simulink library "steadyLevelFlightController_cl"  (R2020a)
settings: Solver=VariableStepAuto  StartTime=0.0  StopTime=10.0  RelTol=1e-3
undefined symbols (not defined in the file or in its folder): env, FLIGHTCONTROLLER, fltCtrl, initializeBussesFromBlock, vhcl
libraries: filteredPIDController_ul x4, ctrlAllocMatrix_cl x1, eulAng2RotMat_ul x1, alphaBeta_ul x1, gnd2TanRotation_ul x1
settings Model: Creator=jldanie5  LastModifiedBy=John Jr
settings DataIOCC: ReturnWorkspaceOutputs=off
settings DebuggingCC: ArithmeticOperatorsInVariantConditions=warning
settings SFSimCC: CustomCodeUndefinedFunction=UseInterfaceOnly

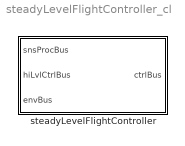
== system steadyLevelFlightController_cl ==
  steadyLevelFlightController : Subsystem  LoadFcn=initializeBussesFromBlock(gcb)  InitFcn=initializeBussesFromBlock(gcb)  StartFcn=initializeBussesFromBlock(gcb)  VariantControl=strcmpi(FLIGHTCONTROLLER,'steadyLevelFlightController')  mask{initPosForInitSStar=vhcl.initPosVecGnd.Value, fluidDensity=env.water.density.Value, pathCtrl=fltCtrl, aeroStruct=vhcl.struct('OCT.aeroSurf')}
      mask prompts: initPosForInitSStar "Initial Position"; fluidDensity "Fluid Density"; pathCtrl "Controller"; aeroStruct "Aerodynamic Structure"
      settings: MinAlgLoopOccurrences=on
      mask DialogControl Container3 Prompt: courseFollow Params
      mask DialogControl Container4 Prompt: setpointToOutput Params

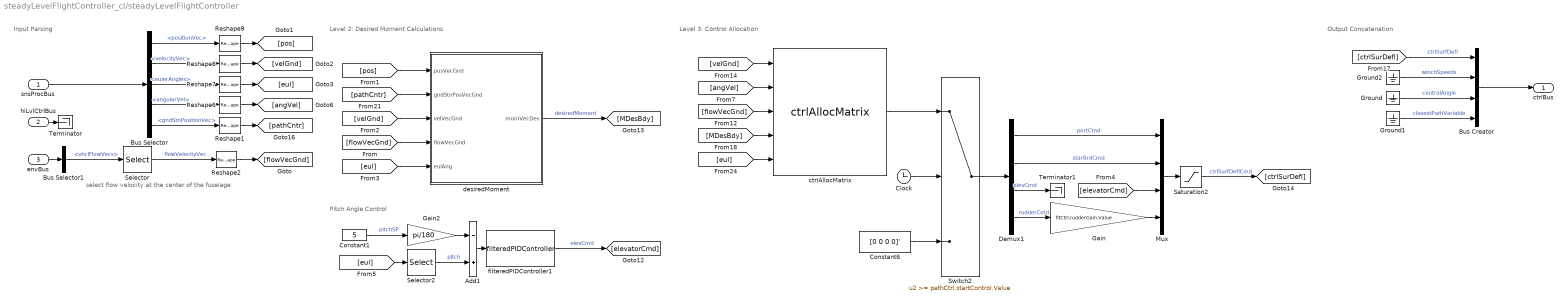
== system steadyLevelFlightController_cl/steadyLevelFlightController ==
  note: select flow velocity at the center of the fuselage
  note: Level 3: Control Allocation
  note: Output Concatenation
  note: Level 2: Desired Moment Calculations
  note: Input Parsing
  note: Pitch Angle Control
  snsProcBus : Inport  OutDataTypeStr=Bus: sensorsProcessingBus
  hiLvlCtrlBus : Inport  Port=2  OutDataTypeStr=Bus: hiLvlCtrlBus
  envBus : Inport  Port=3  OutDataTypeStr=Bus: envBus
  Add1 : Sum  Inputs=-+
  Bus Creator : BusCreator  Inputs=4  OutDataTypeStr=Bus: fltCtrlBus
      settings: InheritFromInputs=off
  Bus Selector : BusSelector  OutputSignals=positionVec,velocityVec,eulerAngles,angularVel,gndStnPositionVec
  Bus Selector1 : BusSelector  OutputSignals=vhclFlowVecs
  Clock : Clock
  Constant1 : Constant  Value=5
  Constant6 : Constant  Value=[0 0 0 0]'
  Demux1 : Demux
  Gain : Gain  Gain=fltCtrl.rudderGain.Value
  Gain2 : Gain  Gain=pi/180
  Ground : Ground
  Ground1 : Ground
  Ground2 : Ground
  Mux : Mux
  Reshape{1..2,6..9} (6 alike) : Reshape  OutputDimensionality=Column vector (2-D)
  Saturation2 : Saturate  UpperLimit=pathCtrl.controlSigMax.upperLimit.Value  LowerLimit=pathCtrl.controlSigMax.lowerLimit.Value
  Selector : Selector  NumberOfDimensions=2  InputPortWidth=3  IndexOptions=Select all,Index vector (dialog)  Indices=[1 3],5  OutputSizes=1,1
  Selector2 : Selector  InputPortWidth=3  IndexOptions=Index vector (dialog)  Indices=2  OutputSizes=1
  Switch2 : Switch  Threshold=pathCtrl.startControl.Value
  Terminator : Terminator
  Terminator1 : Terminator
  ctrlAllocMatrix : ctrlAllocMatrix_cl/ctrlAllocMatrix  aeroStruct=aeroStruct  fluidDensity=fluidDensity
  desiredMoment : Subsystem
  filteredPIDController1 : filteredPIDController_ul/filteredPIDController  kp=pathCtrl.pitchMoment.kp.Value  ki=pathCtrl.pitchMoment.ki.Value  kd=pathCtrl.pitchMoment.kd.Value  Value=pathCtrl.pitchMoment.tau.Value  externalReset=none
  ctrlBus : Outport  OutDataTypeStr=Bus: fltCtrlBus  VectorParamsAs1DForOutWhenUnconnected=off
  wires:
  snsProcBus/1 -> Bus Selector/1
  Bus Selector/2 -> Reshape8/1  "<velocityVec>"
  Bus Selector/1 -> Reshape9/1  "<positionVec>"
  Bus Selector/3 -> Reshape7/1  "<eulerAngles>"
  Bus Creator/1 -> ctrlBus/1
  Ground2/1 -> Bus Creator/2  "winchSpeeds"
  Ground/1 -> Bus Creator/3  "centralAngle"
  Ground1/1 -> Bus Creator/4  "closestPathVariable"
  desiredMoment/1(momVecDes) -> [MDesBdy]  "desiredMoment"
  Bus Selector/4 -> Reshape6/1  "<angularVel>"
  [angVel] -> ctrlAllocMatrix/2
  [velGnd] -> ctrlAllocMatrix/1
  [flowVecGnd] -> ctrlAllocMatrix/3
  Demux1/1 -> Mux/1  "portCmd"
  Demux1/2 -> Mux/2  "starBrdCmd"
  Clock/1 -> Switch2/2
  Switch2/1 -> Demux1/1
  Constant6/1 -> Switch2/3
  [MDesBdy] -> ctrlAllocMatrix/4
  ctrlAllocMatrix/1 -> Switch2/1
  [ctrlSurDefl] -> Bus Creator/1  "ctrlSurfDefl"
  Saturation2/1 -> [ctrlSurDefl]  "ctrlSurfDeflCmd"
  Reshape2/1 -> [flowVecGnd]
  Reshape6/1 -> [angVel]
  Reshape7/1 -> [eul]
  Reshape8/1 -> [velGnd]
  Reshape9/1 -> [pos]
  [eul] -> ctrlAllocMatrix/5
  Selector/1 -> Reshape2/1  "flowVelocityVec"
  envBus/1 -> Bus Selector1/1
  Bus Selector1/1 -> Selector/1  "<vhclFlowVecs>"
  Reshape1/1 -> [pathCntr]
  Bus Selector/5 -> Reshape1/1  "<gndStnPositionVec>"
  [pos] -> desiredMoment/1(posVecGnd)
  [pathCntr] -> desiredMoment/2(gndStnPosVecGnd)
  [velGnd] -> desiredMoment/3(velVecGnd)
  [eul] -> desiredMoment/5(eulAng)
  [flowVecGnd] -> desiredMoment/4(flowVecGnd)
  Gain/1 -> Mux/4
  Demux1/4 -> Gain/1  "rudderCmd"
  hiLvlCtrlBus/1 -> Terminator/1
  Mux/1 -> Saturation2/1
  Demux1/3 -> Terminator1/1  "elevCmd"
  Gain2/1 -> Add1/1
  [eul] -> Selector2/1
  Add1/1 -> filteredPIDController1/1
  Selector2/1 -> Add1/2  "pitch"
  Constant1/1 -> Gain2/1  "pitchSP"
  filteredPIDController1/1 -> [elevatorCmd]  "elevCmd"
  [elevatorCmd] -> Mux/3

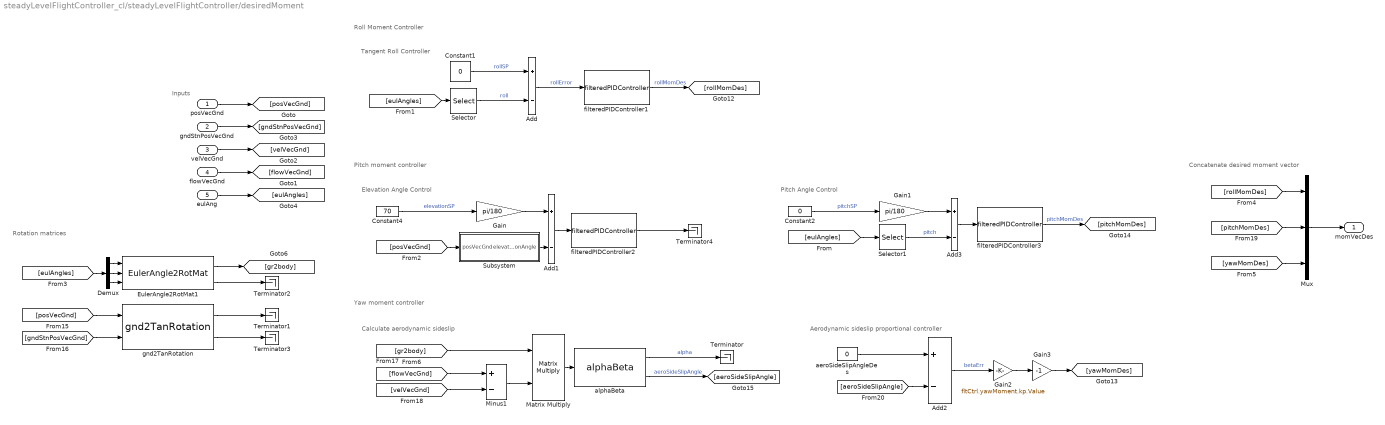
== system steadyLevelFlightController_cl/steadyLevelFlightController/desiredMoment ==
  note: Elevation Angle Control
  note: Inputs
  note: Rotation matrices
  note: Tangent Roll Controller
  note: Concatenate desired moment vector
  note: Aerodynamic sideslip proportional controller
  note: Calculate aerodynamic sideslip
  note: Yaw moment controller
  note: Pitch moment controller
  note: Roll Moment Controller
  note: Pitch Angle Control
  posVecGnd : Inport
  gndStnPosVecGnd : Inport  Port=2
  velVecGnd : Inport  Port=3
  flowVecGnd : Inport  Port=4
  eulAng : Inport  Port=5
  Add{,1..3} (4 alike) : Sum  Inputs=+-
  Constant1 : Constant  Value=0
  Constant2 : Constant  Value=0
  Constant4 : Constant  Value=70
  Demux : Demux  Outputs=3
  EulerAngle2RotMat1 : eulAng2RotMat_ul/EulerAngle2RotMat  SystemSampleTime=-1  Latency=0  AutoFrameSizeCalculation=off
  Gain : Gain  Gain=pi/180
  Gain1 : Gain  Gain=pi/180
  Gain2 : Gain  Gain=fltCtrl.yawMoment.kp.Value
  Gain3 : Gain  Gain=-1
  Matrix Multiply : Product  Multiplication=Matrix(*)
  Minus1 : Sum  Inputs=+-
  Mux : Mux  Inputs=3
  Selector : Selector  InputPortWidth=3  IndexOptions=Index vector (dialog)  Indices=1  OutputSizes=1
  Selector1 : Selector  InputPortWidth=3  IndexOptions=Index vector (dialog)  Indices=2  OutputSizes=1
  Subsystem : Subsystem
  Terminator{,1..4} (5 alike) : Terminator
  aeroSideSlipAngleDes : Constant  Value=0
  alphaBeta : alphaBeta_ul/alphaBeta  SystemSampleTime=-1  Latency=0  AutoFrameSizeCalculation=off
  filteredPIDController1 : filteredPIDController_ul/filteredPIDController  kp=pathCtrl.rollMoment.kp.Value  ki=0  kd=pathCtrl.rollMoment.kd.Value  Value=pathCtrl.rollMoment.tau.Value  externalReset=none
  filteredPIDController2 : filteredPIDController_ul/filteredPIDController  kp=pathCtrl.pitchMoment.kp.Value  ki=pathCtrl.pitchMoment.ki.Value  kd=pathCtrl.pitchMoment.kd.Value  Value=pathCtrl.pitchMoment.tau.Value  externalReset=none
  filteredPIDController3 : filteredPIDController_ul/filteredPIDController  kp=pathCtrl.pitchMoment.kp.Value  ki=pathCtrl.pitchMoment.ki.Value  kd=pathCtrl.pitchMoment.kd.Value  Value=pathCtrl.pitchMoment.tau.Value  externalReset=none
  gnd2TanRotation : gnd2TanRotation_ul/gnd2TanRotation  SystemSampleTime=-1  Latency=0  AutoFrameSizeCalculation=off
  momVecDes : Outport  VectorParamsAs1DForOutWhenUnconnected=off
  wires:
  [aeroSideSlipAngle] -> Add2/2
  [yawMomDes] -> Mux/3
  [rollMomDes] -> Mux/1
  gnd2TanRotation/1 -> Terminator1/1
  gnd2TanRotation/2 -> Terminator3/1
  [gndStnPosVecGnd] -> gnd2TanRotation/2
  [posVecGnd] -> gnd2TanRotation/1
  Constant1/1 -> Add/1  "rollSP"
  gndStnPosVecGnd/1 -> [gndStnPosVecGnd]
  [pitchMomDes] -> Mux/2
  alphaBeta/1 -> Terminator/1  "alpha"
  Gain3/1 -> [yawMomDes]
  Mux/1 -> momVecDes/1
  aeroSideSlipAngleDes/1 -> Add2/1
  Add2/1 -> Gain2/1  "betaErr"
  alphaBeta/2 -> [aeroSideSlipAngle]  "aeroSideSlipAngle"
  Matrix Multiply/1 -> alphaBeta/1
  [gr2body] -> Matrix Multiply/1
  EulerAngle2RotMat1/1 -> [gr2body]
  EulerAngle2RotMat1/2 -> Terminator2/1
  Demux/2 -> EulerAngle2RotMat1/2
  Demux/1 -> EulerAngle2RotMat1/1
  Demux/3 -> EulerAngle2RotMat1/3
  [flowVecGnd] -> Minus1/1
  [velVecGnd] -> Minus1/2
  Minus1/1 -> Matrix Multiply/2
  Gain2/1 -> Gain3/1
  filteredPIDController1/1 -> [rollMomDes]  "rollMomDes"
  flowVecGnd/1 -> [flowVecGnd]
  Add/1 -> filteredPIDController1/1  "rollError"
  velVecGnd/1 -> [velVecGnd]
  posVecGnd/1 -> [posVecGnd]
  Add1/1 -> filteredPIDController2/1
  Constant4/1 -> Gain/1  "elevationSP"
  [posVecGnd] -> Subsystem/1(posVecGnd)
  Subsystem/1(elevationAngle) -> Add1/2
  filteredPIDController2/1 -> Terminator4/1
  eulAng/1 -> [eulAngles]
  [eulAngles] -> Demux/1
  Constant2/1 -> Gain1/1  "pitchSP"
  Add3/1 -> filteredPIDController3/1
  [eulAngles] -> Selector/1
  Selector/1 -> Add/2  "roll"
  [eulAngles] -> Selector1/1
  Selector1/1 -> Add3/2  "pitch"
  filteredPIDController3/1 -> [pitchMomDes]  "pitchMomDes"
  Gain/1 -> Add1/1
  Gain1/1 -> Add3/1

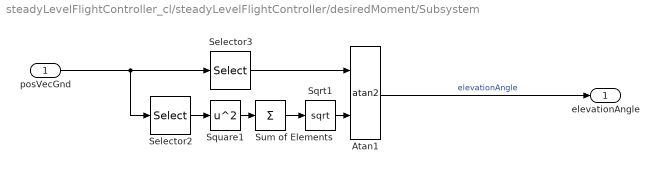
== system steadyLevelFlightController_cl/steadyLevelFlightController/desiredMoment/Subsystem ==
  posVecGnd : Inport
  Atan1 : Trigonometry  Operator=atan2
  Selector2 : Selector  InputPortWidth=3  IndexOptions=Index vector (dialog)  Indices=[1 2]  OutputSizes=1
  Selector3 : Selector  InputPortWidth=3  IndexOptions=Index vector (dialog)  Indices=3  OutputSizes=1
  Sqrt1 : Sqrt  SaturateOnIntegerOverflow=on
  Square1 : Math  Operator=square  SignedPower=on  SaturateOnIntegerOverflow=on
  Sum of Elements : Sum  Inputs=+
  elevationAngle : Outport
  wires:
  Sqrt1/1 -> Atan1/2
  Square1/1 -> Sum of Elements/1
  Selector3/1 -> Atan1/1
  Sum of Elements/1 -> Sqrt1/1
  Atan1/1 -> elevationAngle/1  "elevationAngle"
  Selector2/1 -> Square1/1
  posVecGnd/1 -> Selector2/1, Selector3/1
